simulink subsystem "convolutional_encoder_packet"  (R2024b)
settings: Solver=VariableStepAuto  StartTime=0.0  StopTime=10.0  RelTol=1e-3
values from neighbouring files (symbols this model uses):
  RandomizeSequence = hexToArray(RandomizeSequence,0)    [Full_transmit.m]
  SBLSF = hexToArray(SBLSF,1)    [Full_transmit.m]
libraries: commcnvcod2 x2, simulink x2, commblkintrlv2 x1
settings Model: Creator=SERGIO  LastModifiedBy=SERGIO

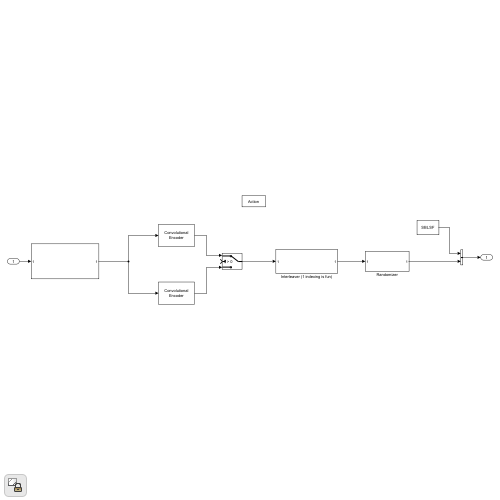
[thumbnail: Simulink's stored preview of the top-level diagram]
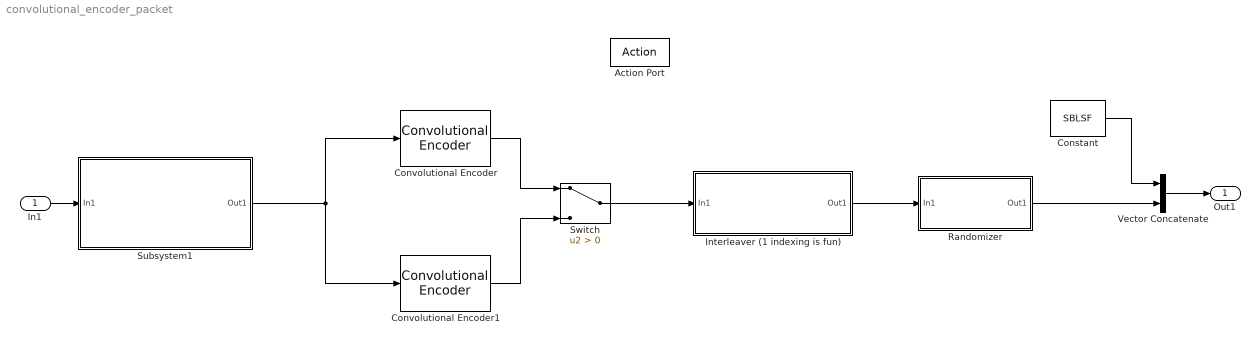
== system convolutional_encoder_packet ==
  In1 : Inport
  Action Port : ActionPort
  Constant : Constant  Value=SBLSF
  Convolutional Encoder : commcnvcod2/Convolutional Encoder  trellis=poly2trellis(5, [23 35])  opMode=Continuous  DelayedResetAction=on  hasIniStPort=off  hasFinStPort=off  usePuncVector=on  punctureVector=Param.Puncture.P3  reset=Unused parameter value
      settings: LibrarySourceBlock=|
      | commhdlcnvcod/Convolutional
      | Encoder
  Convolutional Encoder1 : commcnvcod2/Convolutional Encoder  trellis=poly2trellis(5, [23 35])  opMode=Continuous  DelayedResetAction=on  hasIniStPort=off  hasFinStPort=off  usePuncVector=on  punctureVector=Param.Puncture.P3  reset=Unused parameter value
      settings: LibrarySourceBlock=|
      | commhdlcnvcod/Convolutional
      | Encoder
  Interleaver (1 indexing is fun) : Subsystem
  Randomizer : Subsystem
  Subsystem1 : Subsystem
  Switch : Switch  Criteria=u2 > Threshold  SaturateOnIntegerOverflow=off  InputSameDT=off
  Vector Concatenate : Concatenate
  Out1 : Outport
  wires:
  In1/1 -> Subsystem1/1(In1)
  Randomizer/1(Out1) -> Vector Concatenate/2
  Interleaver (1 indexing is fun)/1(Out1) -> Randomizer/1(In1)
  Subsystem1/1(Out1) -> Convolutional Encoder/1, Convolutional Encoder1/1
  Convolutional Encoder/1 -> Switch/1
  Convolutional Encoder1/1 -> Switch/3
  Switch/1 -> Interleaver (1 indexing is fun)/1(In1)
  Constant/1 -> Vector Concatenate/1
  Vector Concatenate/1 -> Out1/1

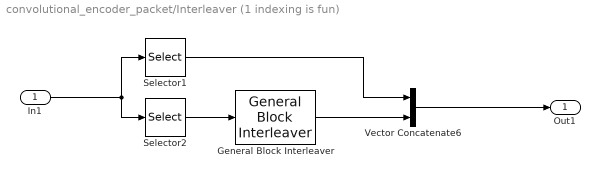
== system convolutional_encoder_packet/Interleaver (1 indexing is fun) ==
  In1 : Inport
  General Block Interleaver : commblkintrlv2/General Block Interleaver  StatePerturbationForJacobian=1.0e-05  permutationVectorSource=Dialog  elements=InterleavingVector
  Selector1 : Selector  IndexOptions=Index vector (dialog)  Indices=[1]  OutputSizes=1
  Selector2 : Selector  IndexOptions=Index vector (dialog)  Indices=[2:368]  OutputSizes=1
  Vector Concatenate6 : Concatenate
  Out1 : Outport
  wires:
  General Block Interleaver/1 -> Vector Concatenate6/2
  Selector1/1 -> Vector Concatenate6/1
  In1/1 -> Selector2/1, Selector1/1
  Selector2/1 -> General Block Interleaver/1
  Vector Concatenate6/1 -> Out1/1

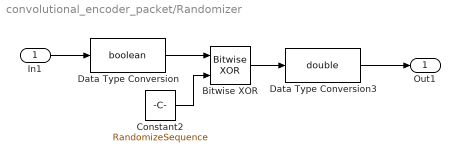
== system convolutional_encoder_packet/Randomizer ==
  In1 : Inport
  Bitwise XOR : simulink/Logic and Bit Operations/Bitwise Operator  logicop=XOR  UseBitMask=off  NumInputPorts=2  BitMask=bin2dec('11011001')  BitMaskRealWorld=Stored Integer
  Constant2 : Constant  Value=RandomizeSequence
  Data Type Conversion : DataTypeConversion  OutDataTypeStr=boolean  SaturateOnIntegerOverflow=off  RndMeth=Floor
  Data Type Conversion3 : DataTypeConversion  OutDataTypeStr=double  SaturateOnIntegerOverflow=off  RndMeth=Floor
  Out1 : Outport
  wires:
  Data Type Conversion/1 -> Bitwise XOR/1
  Data Type Conversion3/1 -> Out1/1
  In1/1 -> Data Type Conversion/1
  Constant2/1 -> Bitwise XOR/2
  Bitwise XOR/1 -> Data Type Conversion3/1

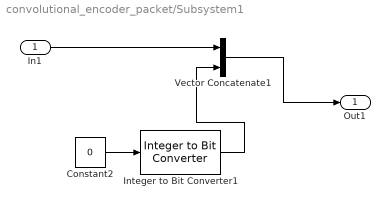
== system convolutional_encoder_packet/Subsystem1 ==
  In1 : Inport
  Constant2 : Constant  Value=0
  Integer to Bit Converter1 : simulink/Logic and Bit Operations/Integer to Bit Converter  nbits=6  signedInputValues=Unsigned  bitOrder=MSB first  outDtype=Inherit via internal rule
  Vector Concatenate1 : Concatenate
  Out1 : Outport
  wires:
  Vector Concatenate1/1 -> Out1/1
  Constant2/1 -> Integer to Bit Converter1/1
  Integer to Bit Converter1/1 -> Vector Concatenate1/2
  In1/1 -> Vector Concatenate1/1
